simulink model "test_qr4_est"  (Simulink 7.0)
settings: Solver=ode45  StartTime=0.0  StopTime=10.0  RelTol=1e-3
libraries: xbsIndex_r4 x1048
(part 1 of 18)
settings Model: Creator=homin  LastModifiedBy=homin
settings DebuggingCC: SaveWithParameterizedLinksMsg=none  SignalResolutionControl=TryResolveAllWithWarning  MultiTaskDSMMsg=warning  MultiTaskCondExecSysMsg=none  StrictBusMsg=None
settings RTWCC: IncludeERTFirstTime=on
settings GRTTargetCC: TargetFcnLib=ansi_tfl_tmw.mat

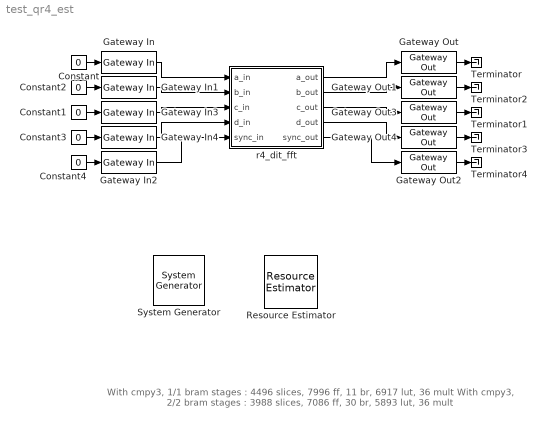
== system test_qr4_est ==
  note: With cmpy3, 1/1 bram stages : 4496 slices, 7996 ff, 11 br, 6917 lut, 36 mult
      | With cmpy3, 2/2 bram stages : 3988 slices, 7086 ff, 30 br, 5893 lut, 36 mult
  " System Generator" : xbsIndex_r4/ System Generator  Tag=genX  SystemSampleTime=-1  xilinxfamily=Virtex2P  part=xc2vp40  speed=-6  package=ff1152  synthesis_tool=XST  clock_wrapper=Clock Enables  directory=./test_qr4_est.netlist  testbench=off  simulink_period=1  sysclk_period=10  dcm_input_clock_period=100  incr_netlist=off  trim_vbits=Everywhere in SubSystem  dbl_ovrd=According to Block Masks  core_generation=According to Block Masks  run_coregen=off  deprecated_control=off  eval_field=0  block_type=sysgen
      settings: block_version=10.1.3
  Constant{,1..4} (5 alike) : Constant  Value=0  OutDataType=sfix(16)  OutScaling=2^0
  Gateway In{,1,3..4} (4 alike) : xbsIndex_r4/Gateway In  arith_type=Unsigned  n_bits=16  bin_pt=0  quantization=Truncate  overflow=Wrap  period=1  dbl_ovrd=off  timing_constraint=None  locs_specified=off  LOCs={}  block_type=gatewayin
      settings: infoedit="Gateway in block.  Converts inputs of type Simulink integer, double and fixed point to  Xilinx fixed point type.<P><P>Hardware notes:  In hardware these blocks become top level input ports."  xl_area=[0 0 0 0 16 0 0]  block_version=10.1.3
  Gateway In2 : xbsIndex_r4/Gateway In  arith_type=Boolean  n_bits=8  bin_pt=6  quantization=Truncate  overflow=Wrap  period=1  dbl_ovrd=off  timing_constraint=None  locs_specified=off  LOCs={}  block_type=gatewayin
      settings: infoedit="Gateway in block.  Converts inputs of type Simulink integer, double and fixed point to  Xilinx fixed point type.<P><P>Hardware notes:  In hardware these blocks become top level input ports."  xl_area=[0 0 0 0 1 0 0]  block_version=10.1.3
  Gateway Out{,1..4} (5 alike) : xbsIndex_r4/Gateway Out  hdl_port=on  timing_constraint=None  locs_specified=off  LOCs={}  block_type=gatewayout
      Gateway Out settings: infoedit="Gateway out block.  Converts Xilinx fixed point inputs into ouputs of type Simulink integer, double, or fixed point.<P><P>Hardware notes:  In hardware these blocks become top level output ports or are discarded, depending on how they are configured."  xl_area=[0 0 0 0 36 0 0]  block_version=10.1.3
      Gateway Out1 settings: infoedit="Gateway out block.  Converts Xilinx fixed point inputs into ouputs of type Simulink integer, double, or fixed point.<P><P>Hardware notes:  In hardware these blocks become top level output ports or are discarded, depending on how they are configured."  xl_area=[0 0 0 0 36 0 0]  block_version=10.1.3
      Gateway Out2 settings: infoedit="Gateway out block.  Converts Xilinx fixed point inputs into ouputs of type Simulink integer, double, or fixed point.<P><P>Hardware notes:  In hardware these blocks become top level output ports or are discarded, depending on how they are configured."  xl_area=[0 0 0 0 1 0 0]  block_version=10.1.3
      Gateway Out3 settings: infoedit="Gateway out block.  Converts Xilinx fixed point inputs into ouputs of type Simulink integer, double, or fixed point.<P><P>Hardware notes:  In hardware these blocks become top level output ports or are discarded, depending on how they are configured."  xl_area=[0 0 0 0 36 0 0]  block_version=10.1.3
      Gateway Out4 settings: infoedit="Gateway out block.  Converts Xilinx fixed point inputs into ouputs of type Simulink integer, double, or fixed point.<P><P>Hardware notes:  In hardware these blocks become top level output ports or are discarded, depending on how they are configured."  xl_area=[0 0 0 0 36 0 0]  block_version=10.1.3
  Resource Estimator : xbsIndex_r4/Resource Estimator  Tag=resEstTag  Slices=4588  FFs=5908  BRAMs=11  LUTs=6917  IOBs=210  EBMs=36  TBUFs=0  xl_use_estimator_area=off  est_options=Estimate  xl_estimator_area=[4496 7996 11 6917 210 36 0]  mrp_directory=./test_qr4_est.netlist  simulink_period=1  block_type=resource_estimator
      settings: AttributesFormatString=Resource Estimator\n%<xl_estimator_area>\n[SL FF BR LUT IO MUL TBUF]  block_version=10.1.3
  Terminator{,1..4} (5 alike) : Terminator
  r4_dit_fft : Subsystem  AncestorBlock=newfft_library/FFT/r4_dit_fft  mask(Quadplex Radix-4 DIT FFT){n_stages=5, n_bits=8, bin_pt=7, shifts=[0], commutator_bram=1, twiddle_bram=1, n_bits_w=9, mult_latency=3, add_latency=1, commute_output=No, output_order=Bit Reversed, show_sbo=on, munge_submasks=DumbDown}
      mask prompts: n_stages "Total Stages"; n_bits "Number of Bits In"; bin_pt "Binary Point In"; shifts "Shifting Schedule"; commutator_bram "Number of Stages Using BRAM for Biplex Commutators (i.e. delays)"; twiddle_bram "Number of Stages Using BRAM for Twiddle Coefficients"; n_bits_w "Twiddle Coefficient Bitwidth"; mult_latency "Multiplier Latency"; add_latency "Adder Latency"; commute_output "Commute Output"; output_order "Output Order"; show_sbo "Show Sub-Block Options"; munge_submasks "Sub-Block Masks"
      mask help: A quadplex radix-4 decimation-in-time Fast Fourier Transform.
      mask init:
      | tic
      | r4_dit_fft_init(gcb, ...
      |   n_stages, ...
      |   n_bits, ...
      |   bin_pt, ...
      |   shifts, ...
      |   commutator_bram, ...
      |   twiddle_bram, ...
      |   n_bits_w, ...
      |   mult_latency, ...
      |   add_latency, ...
      |   commute_output, ...
      |   output_order, ...
      |   lower(get_param(gcb,'munge_submasks')) );
      | disp('r4_dit_fft initialization complete.');
      | toc
      settings: AttributesFormatString=|
      | 1024 points
      | 8_7 r/i in
      | 9_7 twiddles
      mask Help:
      | <pre>
      | Description::
      | 
      | A quadplex radix-4 decimation-in-time Fast Fourier Transform.
      | 
      | The four inputs to the quadplex FFT are independent complex signals (e.g. A, B, C, D).
      | 
      | Without an output commutator, the four outputs of the FFT are commuted such that the
      | a_out signal is really the first quarter of A's transform followed by the first quarter of B's
      | transform, the first quarter of C's transform and the first quarter of D's transform.
      | b_out is really the seconds quarter of A's transform followed by the second quarter of
      | B's transform and so on for the rest of b_out as well as c_out and d_out.
      | 
      | If it is desired to have the four quarters of A's transform follow each other on the
      | same path (and so on for the transforms of B, C, and D), then be sure to check the
      | "Output Commutator" checkbox.  This will result in the four quarters of A's transform
      | (or B's, C's, D's) being in sequential order.  Including the output commutator uses additional
      | resources.
      | 
      | If the Normal Ouput Order option is chosen, the output will be in normal order (though still in
      | commuted quarters if no output commutator is used).  If the "Bit Reversed" Output Order"
      | option is selected, the output quarters (either commuted or not) will each be in bit reversed
      | order (i.e. each quarter of each transform will be in bit reversed output order).   Normal output
      | is easier for humans to work with (especially for testing), but it uses additional resources.
      | Bit reversed output is the implementation's inhernet output order so that option uses no
      | additional resources.
      | 
      | 
      | The number of bits for each real and imaginary component grows by two through this stage.
      | If the bit width grows to exceed 17 bits (when using three real multiplies per complex multiply;
      | 18 bits when using 4 real multiplies per complex multiply), then subsequent stages will
      | comsume more FPGA resources.  A future version will provide an option to limit bit growth.
      | 
      | The number of bits for each real and imaginary component grows by two through each stage.
      | If a stage's input bit width is 17 or less, three embedded multipliers will be used per complex multiply.
      | If a stage's input bit width is 18, four embedded multipliers will be used per complex multiply.
      | If a stage's input bit width exceeds 18, then substantially more embedded multipliers will be used
      | per complex multiply.  Enabling "shifting" in some (or all) stages can limit the bit growth
      | to prevent this.  See the Shifting Schedule parameter for more info.
      | 
      | 
      | Mask Parameters::
      | 
      | Total Stages (n_stages):  The number of total stages in the FFT.
      | The FFT will have 4^n_stages points.
      | 
      | Number of Bits In (n_bits): Specifies the width of the real/imaginary components of ports
      | a_in and b_in.  Assumed equal for both components.  The output bit width will be
      | n_bits+2*n_stages (assuming sum(shifts)==0).
      | 
      | Binary Point In/Out (bin_pt): Specifies the binary point position of the real/imaginary
      | components of ports a_in, b_in, c_in, and d_in.  Assumed equal for both components.
      | 
      | Shifting Schedule (shifts): A vector specifying how many bits to shift by at each stage.
      | Missing values are assumed to be zero; extra values are ignored.
      | 
      | Number of Stages Using BRAM for Biplex Commutators (commutator_bram): Number of stages
      | that will use BRAM for commutator memory.  Remaining stages will use SLR16 elements (slices).
      | 
      | Number of Stages Using BRAM for Twiddle Coefficients (twiddle_bram): Number of stages that
      | will use BRAM for twiddle coeeficient storage.  Remaining stages will use distributed memory
      | (slices).
      | 
      | Twiddle Coefficient Bitwidth (n_bits_w): Specifies the width of the real/imaginary
      | components of the twiddle coefficients.  Assumed equal for both components.
      | 
      | Multiplier Latency (mult_latency): Latency to use for the underlying real multipliers.
      | 
      | Adder Latency (add_latency): Latency to use for the underlying real adders.
      | 
      | Commute Output (commute_output): Popup options for an output commutator.  See decription
      | above for details on the output commutator.  Choices are:
      |     "No" - No output commutator
      |     "Yes (SLR16)" - Include output commutator using SLR16 elements
      |     "Yes (BRAM)" - Include output commutator using BRAM
      | 
      | Output Order (output_order): Popup options for selecting the output order.  See description
      | above for details on the output order.  Choices are:
      |     "Bit Reversed" - Output each half of each transform in bit reversed order.
      |     "Normal" - Output each half of each transform in normal order.
      | </pre>
      mask StyleString: edit,edit,edit,edit,edit,edit,edit,edit,edit,popup(No|Yes (SLR16)|Yes (BRAM)),popup(Bit Reversed|Normal),checkbox,popup(Keep|DumbDown|Unmask)
      mask CallbackString:
      | |||||||||||mvs=get_param(gcb,'MaskVisibilityString');
      | if strcmp(get_param(gcb,'show_sbo'),'on')
      |   onoff='on';
      | else
      |   onoff='off';
      | end
      | mvs=regexprep(mvs,'o[nf]*$',onoff);
      | set_param(gcb,'MaskVisibilityString',mvs);
      | |
  wires:
  Gateway In/1 -> r4_dit_fft/1(a_in)
  r4_dit_fft/1(a_out) -> Gateway Out/1
  Gateway In1/1 -> r4_dit_fft/2(b_in)
  Gateway In2/1 -> r4_dit_fft/5(sync_in)
  r4_dit_fft/2(b_out) -> Gateway Out1/1
  r4_dit_fft/5(sync_out) -> Gateway Out2/1
  Constant/1 -> Gateway In/1
  Constant2/1 -> Gateway In1/1
  Constant4/1 -> Gateway In2/1
  Gateway Out/1 -> Terminator/1
  Gateway Out1/1 -> Terminator2/1
  Gateway Out2/1 -> Terminator4/1
  Gateway In3/1 -> r4_dit_fft/3(c_in)
  Gateway In4/1 -> r4_dit_fft/4(d_in)
  Constant1/1 -> Gateway In3/1
  Constant3/1 -> Gateway In4/1
  r4_dit_fft/3(c_out) -> Gateway Out3/1
  r4_dit_fft/4(d_out) -> Gateway Out4/1
  Gateway Out3/1 -> Terminator1/1
  Gateway Out4/1 -> Terminator3/1

== system test_qr4_est/r4_dit_fft ==
  a_in : Inport  OutDataType=sfix(16)  OutScaling=2^0
  b_in : Inport  Port=2  OutDataType=sfix(16)  OutScaling=2^0
  c_in : Inport  Port=3  OutDataType=sfix(16)  OutScaling=2^0
  d_in : Inport  Port=4  OutDataType=sfix(16)  OutScaling=2^0
  sync_in : Inport  Port=5  OutDataType=sfix(16)  OutScaling=2^0
  r4_dit_stage_1 : Subsystem  mask(Radix-4 DIT FFT Stage){n_stages=5, cur_stage=1, n_bits=8, bin_pt=7, shift=0, commutator_bram=on, twiddle_bram=off, n_bits_w=9, mult_latency=3, add_latency=1}
      mask prompts: n_stages "Total Stages (4^N points)"; cur_stage "Current Stage"; n_bits "Number of Bits In"; bin_pt "Binary Point In"; shift "Shift Bits"; commutator_bram "Use BRAM for Quadplex Commutator"; twiddle_bram "Use BRAM for Twiddle Coefficients"; n_bits_w "Twiddle Coefficient Bitwidth"; mult_latency "Multiplier Latency"; add_latency "Adder Latency"
      mask help: A radix-4 decimation-in-time Fast Fourier Transform stage.
      settings: AttributesFormatString=|
      | stage 1 of 5
      | delay bram
      | twiddle dist
      | shift 0
      mask Help:
      | <pre>
      | Description::
      | 
      | A radix-4 decimation-in-time Fast Fourier Transform stage.
      | 
      | This radix-4 decimation-in-time FFT stage is designed to be daisy chained together
      | to form a multi-stage FFT.  The resulting FFT will have (4^n_stages) points.
      | 
      | The four inputs to the chain are independent complex signals (e.g. A, B, C, and D).
      | 
      | The four outputs of the last stage of the chain are commuted such that the a_out signal is really
      | the first quarter of A's transform followed by the first quarter of B's transform, the first quarter
      | of C's transform and the first quarter of D's transform.  b_out is really the seconds quarter of
      | A's transform followed by the second quarter of B's transform and so on for the rest of b_out
      | as well as c_out and d_out.  Each quarter is in bit-reversed order.
      | 
      | If it is desired to have the four quarters of A's transform follow each other on the
      | same path (and so on for the transforms of B, C, and D), then a_out and b_out can
      | be fed through a quadplex_commutator with block size 4^n_stages.  This will result
      | in the four quarters of A's transform (or B's, C's, D's) being in sequential order,
      | but note that each quarter of A's transform will still remain in bit-reversed order
      | (i.e. each output is bit-reversed in quarterss; it is not bit reversed in its entirety).
      | 
      | The number of bits for each real and imaginary component grows by two through this stage.
      | If the input bit width is 17 or less, three embedded multipliers will be used per complex multiply.
      | If the input bit width is 18, four embedded multipliers will be used per complex multiply.
      | If the input bit width exceeds 18, then substantially more embedded multipliers will be used
      | per complex multiply.  Enabling "shifting" in some (or all) stages can limit the bit growth
      | to prevent this.
      | 
      | Mask Parameters::
      | 
      | Total Stages (n_stages):  The number of total stages in the FFT.
      | The FFT will have 4^n_stages points.
      | 
      | Current Stage (cur_stage):  The number of the current stage.  Note that stages are counted
      | from 1 to n_stages for DIT (i.e. cur_stage==1 for the first stage).
      | 
      | Number of Bits In (n_bits): Specifies the width of the real/imaginary components of ports
      | a_in and b_in.  Assumed equal for both components.  The real/imaginary components of
      | oorts a_out and b_out will be one bit wider.
      | 
      | Binary Point In (bin_pt): Specifies the binary point position of the real/imaginary
      | components of ports a_in and b_in.  Assumed equal for both components.
      | 
      | Shift Bits (shift): Specifies how many bits to shift (down) by.  A positive value causes
      | the specified number of least significant bits to be dropped.  Usually zero or positive values
      | are used to permit or limit bit growth, but negative values can be used to induce bit growth.
      | 
      | Use BRAM for Biplex Commutator (commutator_bram): Check this checkbox to implement
      | the biplex commutator using BRAM.  If unchecked, the biplex commutator will be implemented
      | using SLR16 elements (i.e. slices).
      | 
      | Use BRAM for Twiddle Coefficients (twiddle_bram): Check this checkbox to store twiddle
      | coefficients in BRAM.  If unchecked, the twiddle coefficients will be sored in distributed
      | memory (i.e. slices).
      | 
      | Twiddle Coefficient Bitwidth (n_bits_w): Specifies the width of the real/imaginary
      | components of the twiddle coefficients.  Assumed equal for both components.
      | 
      | Multiplier Latency (mult_latency): Latency to use for the underlying real multipliers.
      | 
      | Adder Latency (add_latency): Latency to use for the underlying real adders.
      | </pre>
  r4_dit_stage_2 : Subsystem  mask(Radix-4 DIT FFT Stage){n_stages=5, cur_stage=2, n_bits=10, bin_pt=7, shift=0, commutator_bram=off, twiddle_bram=off, n_bits_w=9, mult_latency=3, add_latency=1}
      mask prompts: n_stages "Total Stages (4^N points)"; cur_stage "Current Stage"; n_bits "Number of Bits In"; bin_pt "Binary Point In"; shift "Shift Bits"; commutator_bram "Use BRAM for Quadplex Commutator"; twiddle_bram "Use BRAM for Twiddle Coefficients"; n_bits_w "Twiddle Coefficient Bitwidth"; mult_latency "Multiplier Latency"; add_latency "Adder Latency"
      mask help: A radix-4 decimation-in-time Fast Fourier Transform stage.
      settings: AttributesFormatString=|
      | stage 2 of 5
      | delay slr
      | twiddle dist
      | shift 0
      mask Help:
      | <pre>
      | Description::
      | 
      | A radix-4 decimation-in-time Fast Fourier Transform stage.
      | 
      | This radix-4 decimation-in-time FFT stage is designed to be daisy chained together
      | to form a multi-stage FFT.  The resulting FFT will have (4^n_stages) points.
      | 
      | The four inputs to the chain are independent complex signals (e.g. A, B, C, and D).
      | 
      | The four outputs of the last stage of the chain are commuted such that the a_out signal is really
      | the first quarter of A's transform followed by the first quarter of B's transform, the first quarter
      | of C's transform and the first quarter of D's transform.  b_out is really the seconds quarter of
      | A's transform followed by the second quarter of B's transform and so on for the rest of b_out
      | as well as c_out and d_out.  Each quarter is in bit-reversed order.
      | 
      | If it is desired to have the four quarters of A's transform follow each other on the
      | same path (and so on for the transforms of B, C, and D), then a_out and b_out can
      | be fed through a quadplex_commutator with block size 4^n_stages.  This will result
      | in the four quarters of A's transform (or B's, C's, D's) being in sequential order,
      | but note that each quarter of A's transform will still remain in bit-reversed order
      | (i.e. each output is bit-reversed in quarterss; it is not bit reversed in its entirety).
      | 
      | The number of bits for each real and imaginary component grows by two through this stage.
      | If the input bit width is 17 or less, three embedded multipliers will be used per complex multiply.
      | If the input bit width is 18, four embedded multipliers will be used per complex multiply.
      | If the input bit width exceeds 18, then substantially more embedded multipliers will be used
      | per complex multiply.  Enabling "shifting" in some (or all) stages can limit the bit growth
      | to prevent this.
      | 
      | Mask Parameters::
      | 
      | Total Stages (n_stages):  The number of total stages in the FFT.
      | The FFT will have 4^n_stages points.
      | 
      | Current Stage (cur_stage):  The number of the current stage.  Note that stages are counted
      | from 1 to n_stages for DIT (i.e. cur_stage==1 for the first stage).
      | 
      | Number of Bits In (n_bits): Specifies the width of the real/imaginary components of ports
      | a_in and b_in.  Assumed equal for both components.  The real/imaginary components of
      | oorts a_out and b_out will be one bit wider.
      | 
      | Binary Point In (bin_pt): Specifies the binary point position of the real/imaginary
      | components of ports a_in and b_in.  Assumed equal for both components.
      | 
      | Shift Bits (shift): Specifies how many bits to shift (down) by.  A positive value causes
      | the specified number of least significant bits to be dropped.  Usually zero or positive values
      | are used to permit or limit bit growth, but negative values can be used to induce bit growth.
      | 
      | Use BRAM for Biplex Commutator (commutator_bram): Check this checkbox to implement
      | the biplex commutator using BRAM.  If unchecked, the biplex commutator will be implemented
      | using SLR16 elements (i.e. slices).
      | 
      | Use BRAM for Twiddle Coefficients (twiddle_bram): Check this checkbox to store twiddle
      | coefficients in BRAM.  If unchecked, the twiddle coefficients will be sored in distributed
      | memory (i.e. slices).
      | 
      | Twiddle Coefficient Bitwidth (n_bits_w): Specifies the width of the real/imaginary
      | components of the twiddle coefficients.  Assumed equal for both components.
      | 
      | Multiplier Latency (mult_latency): Latency to use for the underlying real multipliers.
      | 
      | Adder Latency (add_latency): Latency to use for the underlying real adders.
      | </pre>
  r4_dit_stage_3 : Subsystem  mask(Radix-4 DIT FFT Stage){n_stages=5, cur_stage=3, n_bits=12, bin_pt=7, shift=0, commutator_bram=off, twiddle_bram=off, n_bits_w=9, mult_latency=3, add_latency=1}
      mask prompts: n_stages "Total Stages (4^N points)"; cur_stage "Current Stage"; n_bits "Number of Bits In"; bin_pt "Binary Point In"; shift "Shift Bits"; commutator_bram "Use BRAM for Quadplex Commutator"; twiddle_bram "Use BRAM for Twiddle Coefficients"; n_bits_w "Twiddle Coefficient Bitwidth"; mult_latency "Multiplier Latency"; add_latency "Adder Latency"
      mask help: A radix-4 decimation-in-time Fast Fourier Transform stage.
      settings: AttributesFormatString=|
      | stage 3 of 5
      | delay slr
      | twiddle dist
      | shift 0
      mask Help:
      | <pre>
      | Description::
      | 
      | A radix-4 decimation-in-time Fast Fourier Transform stage.
      | 
      | This radix-4 decimation-in-time FFT stage is designed to be daisy chained together
      | to form a multi-stage FFT.  The resulting FFT will have (4^n_stages) points.
      | 
      | The four inputs to the chain are independent complex signals (e.g. A, B, C, and D).
      | 
      | The four outputs of the last stage of the chain are commuted such that the a_out signal is really
      | the first quarter of A's transform followed by the first quarter of B's transform, the first quarter
      | of C's transform and the first quarter of D's transform.  b_out is really the seconds quarter of
      | A's transform followed by the second quarter of B's transform and so on for the rest of b_out
      | as well as c_out and d_out.  Each quarter is in bit-reversed order.
      | 
      | If it is desired to have the four quarters of A's transform follow each other on the
      | same path (and so on for the transforms of B, C, and D), then a_out and b_out can
      | be fed through a quadplex_commutator with block size 4^n_stages.  This will result
      | in the four quarters of A's transform (or B's, C's, D's) being in sequential order,
      | but note that each quarter of A's transform will still remain in bit-reversed order
      | (i.e. each output is bit-reversed in quarterss; it is not bit reversed in its entirety).
      | 
      | The number of bits for each real and imaginary component grows by two through this stage.
      | If the input bit width is 17 or less, three embedded multipliers will be used per complex multiply.
      | If the input bit width is 18, four embedded multipliers will be used per complex multiply.
      | If the input bit width exceeds 18, then substantially more embedded multipliers will be used
      | per complex multiply.  Enabling "shifting" in some (or all) stages can limit the bit growth
      | to prevent this.
      | 
      | Mask Parameters::
      | 
      | Total Stages (n_stages):  The number of total stages in the FFT.
      | The FFT will have 4^n_stages points.
      | 
      | Current Stage (cur_stage):  The number of the current stage.  Note that stages are counted
      | from 1 to n_stages for DIT (i.e. cur_stage==1 for the first stage).
      | 
      | Number of Bits In (n_bits): Specifies the width of the real/imaginary components of ports
      | a_in and b_in.  Assumed equal for both components.  The real/imaginary components of
      | oorts a_out and b_out will be one bit wider.
      | 
      | Binary Point In (bin_pt): Specifies the binary point position of the real/imaginary
      | components of ports a_in and b_in.  Assumed equal for both components.
      | 
      | Shift Bits (shift): Specifies how many bits to shift (down) by.  A positive value causes
      | the specified number of least significant bits to be dropped.  Usually zero or positive values
      | are used to permit or limit bit growth, but negative values can be used to induce bit growth.
      | 
      | Use BRAM for Biplex Commutator (commutator_bram): Check this checkbox to implement
      | the biplex commutator using BRAM.  If unchecked, the biplex commutator will be implemented
      | using SLR16 elements (i.e. slices).
      | 
      | Use BRAM for Twiddle Coefficients (twiddle_bram): Check this checkbox to store twiddle
      | coefficients in BRAM.  If unchecked, the twiddle coefficients will be sored in distributed
      | memory (i.e. slices).
      | 
      | Twiddle Coefficient Bitwidth (n_bits_w): Specifies the width of the real/imaginary
      | components of the twiddle coefficients.  Assumed equal for both components.
      | 
      | Multiplier Latency (mult_latency): Latency to use for the underlying real multipliers.
      | 
      | Adder Latency (add_latency): Latency to use for the underlying real adders.
      | </pre>
  r4_dit_stage_4 : Subsystem  mask(Radix-4 DIT FFT Stage){n_stages=5, cur_stage=4, n_bits=14, bin_pt=7, shift=0, commutator_bram=off, twiddle_bram=off, n_bits_w=9, mult_latency=3, add_latency=1}
      mask prompts: n_stages "Total Stages (4^N points)"; cur_stage "Current Stage"; n_bits "Number of Bits In"; bin_pt "Binary Point In"; shift "Shift Bits"; commutator_bram "Use BRAM for Quadplex Commutator"; twiddle_bram "Use BRAM for Twiddle Coefficients"; n_bits_w "Twiddle Coefficient Bitwidth"; mult_latency "Multiplier Latency"; add_latency "Adder Latency"
      mask help: A radix-4 decimation-in-time Fast Fourier Transform stage.
      settings: AttributesFormatString=|
      | stage 4 of 5
      | delay slr
      | twiddle dist
      | shift 0
      mask Help:
      | <pre>
      | Description::
      | 
      | A radix-4 decimation-in-time Fast Fourier Transform stage.
      | 
      | This radix-4 decimation-in-time FFT stage is designed to be daisy chained together
      | to form a multi-stage FFT.  The resulting FFT will have (4^n_stages) points.
      | 
      | The four inputs to the chain are independent complex signals (e.g. A, B, C, and D).
      | 
      | The four outputs of the last stage of the chain are commuted such that the a_out signal is really
      | the first quarter of A's transform followed by the first quarter of B's transform, the first quarter
      | of C's transform and the first quarter of D's transform.  b_out is really the seconds quarter of
      | A's transform followed by the second quarter of B's transform and so on for the rest of b_out
      | as well as c_out and d_out.  Each quarter is in bit-reversed order.
      | 
      | If it is desired to have the four quarters of A's transform follow each other on the
      | same path (and so on for the transforms of B, C, and D), then a_out and b_out can
      | be fed through a quadplex_commutator with block size 4^n_stages.  This will result
      | in the four quarters of A's transform (or B's, C's, D's) being in sequential order,
      | but note that each quarter of A's transform will still remain in bit-reversed order
      | (i.e. each output is bit-reversed in quarterss; it is not bit reversed in its entirety).
      | 
      | The number of bits for each real and imaginary component grows by two through this stage.
      | If the input bit width is 17 or less, three embedded multipliers will be used per complex multiply.
      | If the input bit width is 18, four embedded multipliers will be used per complex multiply.
      | If the input bit width exceeds 18, then substantially more embedded multipliers will be used
      | per complex multiply.  Enabling "shifting" in some (or all) stages can limit the bit growth
      | to prevent this.
      | 
      | Mask Parameters::
      | 
      | Total Stages (n_stages):  The number of total stages in the FFT.
      | The FFT will have 4^n_stages points.
      | 
      | Current Stage (cur_stage):  The number of the current stage.  Note that stages are counted
      | from 1 to n_stages for DIT (i.e. cur_stage==1 for the first stage).
      | 
      | Number of Bits In (n_bits): Specifies the width of the real/imaginary components of ports
      | a_in and b_in.  Assumed equal for both components.  The real/imaginary components of
      | oorts a_out and b_out will be one bit wider.
      | 
      | Binary Point In (bin_pt): Specifies the binary point position of the real/imaginary
      | components of ports a_in and b_in.  Assumed equal for both components.
      | 
      | Shift Bits (shift): Specifies how many bits to shift (down) by.  A positive value causes
      | the specified number of least significant bits to be dropped.  Usually zero or positive values
      | are used to permit or limit bit growth, but negative values can be used to induce bit growth.
      | 
      | Use BRAM for Biplex Commutator (commutator_bram): Check this checkbox to implement
      | the biplex commutator using BRAM.  If unchecked, the biplex commutator will be implemented
      | using SLR16 elements (i.e. slices).
      | 
      | Use BRAM for Twiddle Coefficients (twiddle_bram): Check this checkbox to store twiddle
      | coefficients in BRAM.  If unchecked, the twiddle coefficients will be sored in distributed
      | memory (i.e. slices).
      | 
      | Twiddle Coefficient Bitwidth (n_bits_w): Specifies the width of the real/imaginary
      | components of the twiddle coefficients.  Assumed equal for both components.
      | 
      | Multiplier Latency (mult_latency): Latency to use for the underlying real multipliers.
      | 
      | Adder Latency (add_latency): Latency to use for the underlying real adders.
      | </pre>
  r4_dit_stage_5 : Subsystem  mask(Radix-4 DIT FFT Stage){n_stages=5, cur_stage=5, n_bits=16, bin_pt=7, shift=0, commutator_bram=off, twiddle_bram=on, n_bits_w=9, mult_latency=3, add_latency=1}
      mask prompts: n_stages "Total Stages (4^N points)"; cur_stage "Current Stage"; n_bits "Number of Bits In"; bin_pt "Binary Point In"; shift "Shift Bits"; commutator_bram "Use BRAM for Quadplex Commutator"; twiddle_bram "Use BRAM for Twiddle Coefficients"; n_bits_w "Twiddle Coefficient Bitwidth"; mult_latency "Multiplier Latency"; add_latency "Adder Latency"
      mask help: A radix-4 decimation-in-time Fast Fourier Transform stage.
      settings: AttributesFormatString=|
      | stage 5 of 5
      | delay slr
      | twiddle bram
      | shift 0
      mask Help:
      | <pre>
      | Description::
      | 
      | A radix-4 decimation-in-time Fast Fourier Transform stage.
      | 
      | This radix-4 decimation-in-time FFT stage is designed to be daisy chained together
      | to form a multi-stage FFT.  The resulting FFT will have (4^n_stages) points.
      | 
      | The four inputs to the chain are independent complex signals (e.g. A, B, C, and D).
      | 
      | The four outputs of the last stage of the chain are commuted such that the a_out signal is really
      | the first quarter of A's transform followed by the first quarter of B's transform, the first quarter
      | of C's transform and the first quarter of D's transform.  b_out is really the seconds quarter of
      | A's transform followed by the second quarter of B's transform and so on for the rest of b_out
      | as well as c_out and d_out.  Each quarter is in bit-reversed order.
      | 
      | If it is desired to have the four quarters of A's transform follow each other on the
      | same path (and so on for the transforms of B, C, and D), then a_out and b_out can
      | be fed through a quadplex_commutator with block size 4^n_stages.  This will result
      | in the four quarters of A's transform (or B's, C's, D's) being in sequential order,
      | but note that each quarter of A's transform will still remain in bit-reversed order
      | (i.e. each output is bit-reversed in quarterss; it is not bit reversed in its entirety).
      | 
      | The number of bits for each real and imaginary component grows by two through this stage.
      | If the input bit width is 17 or less, three embedded multipliers will be used per complex multiply.
      | If the input bit width is 18, four embedded multipliers will be used per complex multiply.
      | If the input bit width exceeds 18, then substantially more embedded multipliers will be used
      | per complex multiply.  Enabling "shifting" in some (or all) stages can limit the bit growth
      | to prevent this.
      | 
      | Mask Parameters::
      | 
      | Total Stages (n_stages):  The number of total stages in the FFT.
      | The FFT will have 4^n_stages points.
      | 
      | Current Stage (cur_stage):  The number of the current stage.  Note that stages are counted
      | from 1 to n_stages for DIT (i.e. cur_stage==1 for the first stage).
      | 
      | Number of Bits In (n_bits): Specifies the width of the real/imaginary components of ports
      | a_in and b_in.  Assumed equal for both components.  The real/imaginary components of
      | oorts a_out and b_out will be one bit wider.
      | 
      | Binary Point In (bin_pt): Specifies the binary point position of the real/imaginary
      | components of ports a_in and b_in.  Assumed equal for both components.
      | 
      | Shift Bits (shift): Specifies how many bits to shift (down) by.  A positive value causes
      | the specified number of least significant bits to be dropped.  Usually zero or positive values
      | are used to permit or limit bit growth, but negative values can be used to induce bit growth.
      | 
      | Use BRAM for Biplex Commutator (commutator_bram): Check this checkbox to implement
      | the biplex commutator using BRAM.  If unchecked, the biplex commutator will be implemented
      | using SLR16 elements (i.e. slices).
      | 
      | Use BRAM for Twiddle Coefficients (twiddle_bram): Check this checkbox to store twiddle
      | coefficients in BRAM.  If unchecked, the twiddle coefficients will be sored in distributed
      | memory (i.e. slices).
      | 
      | Twiddle Coefficient Bitwidth (n_bits_w): Specifies the width of the real/imaginary
      | components of the twiddle coefficients.  Assumed equal for both components.
      | 
      | Multiplier Latency (mult_latency): Latency to use for the underlying real multipliers.
      | 
      | Adder Latency (add_latency): Latency to use for the underlying real adders.
      | </pre>
  a_out : Outport  OutDataType=sfix(16)  OutScaling=2^0
  b_out : Outport  Port=2  OutDataType=sfix(16)  OutScaling=2^0
  c_out : Outport  Port=3  OutDataType=sfix(16)  OutScaling=2^0
  d_out : Outport  Port=4  OutDataType=sfix(16)  OutScaling=2^0
  sync_out : Outport  Port=5  OutDataType=sfix(16)  OutScaling=2^0
  wires:
  a_in/1 -> r4_dit_stage_1/1(a_in)
  b_in/1 -> r4_dit_stage_1/2(b_in)
  c_in/1 -> r4_dit_stage_1/3(c_in)
  d_in/1 -> r4_dit_stage_1/4(d_in)
  sync_in/1 -> r4_dit_stage_1/5(sync_in)
  r4_dit_stage_1/1(a_out) -> r4_dit_stage_2/1(a_in)
  r4_dit_stage_1/2(b_out) -> r4_dit_stage_2/2(b_in)
  r4_dit_stage_1/3(c_out) -> r4_dit_stage_2/3(c_in)
  r4_dit_stage_1/4(d_out) -> r4_dit_stage_2/4(d_in)
  r4_dit_stage_1/5(sync_out) -> r4_dit_stage_2/5(sync_in)
  r4_dit_stage_2/1(a_out) -> r4_dit_stage_3/1(a_in)
  r4_dit_stage_2/2(b_out) -> r4_dit_stage_3/2(b_in)
  r4_dit_stage_2/3(c_out) -> r4_dit_stage_3/3(c_in)
  r4_dit_stage_2/4(d_out) -> r4_dit_stage_3/4(d_in)
  r4_dit_stage_2/5(sync_out) -> r4_dit_stage_3/5(sync_in)
  r4_dit_stage_3/1(a_out) -> r4_dit_stage_4/1(a_in)
  r4_dit_stage_3/2(b_out) -> r4_dit_stage_4/2(b_in)
  r4_dit_stage_3/3(c_out) -> r4_dit_stage_4/3(c_in)
  r4_dit_stage_3/4(d_out) -> r4_dit_stage_4/4(d_in)
  r4_dit_stage_3/5(sync_out) -> r4_dit_stage_4/5(sync_in)
  r4_dit_stage_4/1(a_out) -> r4_dit_stage_5/1(a_in)
  r4_dit_stage_4/2(b_out) -> r4_dit_stage_5/2(b_in)
  r4_dit_stage_4/3(c_out) -> r4_dit_stage_5/3(c_in)
  r4_dit_stage_4/4(d_out) -> r4_dit_stage_5/4(d_in)
  r4_dit_stage_4/5(sync_out) -> r4_dit_stage_5/5(sync_in)
  r4_dit_stage_5/1(a_out) -> a_out/1
  r4_dit_stage_5/3(c_out) -> b_out/1
  r4_dit_stage_5/2(b_out) -> c_out/1
  r4_dit_stage_5/4(d_out) -> d_out/1
  r4_dit_stage_5/5(sync_out) -> sync_out/1

== system test_qr4_est/r4_dit_fft/r4_dit_stage_1 ==
  a_in : Inport  OutDataType=sfix(16)  OutScaling=2^0
  b_in : Inport  Port=2  OutDataType=sfix(16)  OutScaling=2^0
  c_in : Inport  Port=3  OutDataType=sfix(16)  OutScaling=2^0
  d_in : Inport  Port=4  OutDataType=sfix(16)  OutScaling=2^0
  sync_in : Inport  Port=5  OutDataType=sfix(16)  OutScaling=2^0
  quadplex_commutator : Subsystem  mask(Quadplex Commutator){log4_size=5, n_bits=8, use_bram=on}
      mask prompts: log4_size "Log4 Block Size"; n_bits "Bit Width"; use_bram "Use BRAM"
      mask help: The quadplex commutator performs a "quarter-blockwise" commutation of the four inputs. A "block" is 4^log4_size consecutive samples (i.e. always a power of 4). sync_in precedes the first data input sample by one clock cycle. Overall latency from sync_in to sync_out is 2^(log4_size)+2^(log4_size-1)+2.
      settings: AttributesFormatString=|
      | size = 1024
      | 4/4 bram
      mask Help:
      | <pre>
      | Description::
      | 
      | The quadplex commutator performs a "quarter-blockwise" commutation of the four inputs.
      | A "block" is 4^log4_size consecutive samples (i.e. always a power of 4).
      | 
      | sync_in precedes the first data input sample by one clock cycle.
      | sync_out precedes the corresponding output sample by one clock cycle.
      | Overall latency from sync_in to sync_out is 2^(log4_size)+2^(log4_size-1)+2.
      | 
      | Mask Parameters::
      | 
      | Log4 Block Size (log4_size): The base-4 logarithm of the length of one complete input block.
      | This MUST be an integer because the current implementation requires that
      | the input block size MUST be a power of 4.  (aka "N")
      | 
      | Bit Width (n_bits): Specifies the width of the real/imaginary components.
      | Width of each component is assumed equal.
      | 
      | Use BRAM (use_bram): Check this checkbox to implement the internal delays using BRAM.
      | If unchecked, the internal delays will be implemented using SLR16 elements.
      | </pre>
  r4_butterfly : Subsystem  mask(Radix-4 Butterfly){n_bits=8, shift=0, quantization=Truncate, add_latency=1}
      mask prompts: n_bits "Bit Width In"; shift "Shift Bits"; add_latency "Adder Latency"
      mask help: The radix-4 butterfly performs a 4 point FFT on its four inputs (a_in,b_in,c_in,d_in), which are assumed to be in normal order. Its ouputs (a_out,b_out,c_out,d_out) are in bit-reversed order (despite the lexigraphical ordering of the output port names).
      settings: AttributesFormatString=shift 0
      mask Help:
      | <pre>
      | Description::
      | 
      | The radix-4 butterfly performs a 4 point FFT on its four inputs (a_in,b_in,c_in,d_in),
      | which are assumed to be in normal order.  Its ouputs (a_out,b_out,c_out,d_out) are
      | in bit-reversed order (despite the lexigraphical ordering of the output port names).
      | 
      | The outputs are two bits wider than the inputs.
      | The output precision (i.e. the number of fractional bits) stays the same.
      | 
      | Mask Parameters::
      | 
      | Bit Width In (n_bits): Specifies the width of the real/imaginary components.
      | Width of each component is assumed equal.
      | 
      | Shift Bits (shift): Specifies how many bits to shift (down) by.  A positive value causes
      | the specified number of least significant bits to be dropped.  Usually zero or positive values
      | are used to permit or limit bit growth, but negative values can be used to induce bit growth.
      | 
      | Quantization (quantization): Specifies quantization handling (when shift bits > 0).
      | 
      | Adder Latency (add_latency): Latency to use for the underlying real adders.
      | </pre>
      mask StyleString: edit,edit,popup(Truncate|Round  (unbiased: +/- Inf)|Round  (unbiased: Even Values)),edit
  r4_twiddle : Subsystem
      mask Type: Radix-4 Stage-1 Twiddle Stage
      mask Description: A stage-1 twiddle stage for radix-4 Fast Fourier Transforms. Since there are no twiddles in stage 1 of an FFT, this is just a dummy placeholder block that passes its inputs through to its outputs.    Since it is a no-op, its use is completely optional.
      mask Help:
      | <pre>
      | Description::
      | 
      | A stage-1 twiddle stage for radix-4 Fast Fourier Transforms.
      | 
      | Since there are no twiddles in stage 1 of an FFT, this is just a dummy placeholder
      | block that passes its inputs through to its outputs.
      | 
      | Since it is a no-op, its use is completely optional.
      | 
      | Note that stages are counted from 1 to n_stages for DIT (i.e. cur_stage==1 for the first stage)
      | and n_stages to 1for DIF (i.e. cur_stage==1 for the last stage).  Therefore, this block, if used,
      | should be the first twiddle stage of a DIT FFT or the last twiddle stage of a DIF FFT.
      | 
      | Mask Parameters::
      | 
      | (N/A)
  a_out : Outport  OutDataType=sfix(16)  OutScaling=2^0
  b_out : Outport  Port=2  OutDataType=sfix(16)  OutScaling=2^0
  c_out : Outport  Port=3  OutDataType=sfix(16)  OutScaling=2^0
  d_out : Outport  Port=4  OutDataType=sfix(16)  OutScaling=2^0
  sync_out : Outport  Port=5  OutDataType=sfix(16)  OutScaling=2^0
  wires:
  r4_butterfly/5(sync_out) -> sync_out/1
  r4_butterfly/4(d_out) -> d_out/1
  r4_butterfly/3(c_out) -> c_out/1
  r4_butterfly/2(b_out) -> b_out/1
  r4_butterfly/1(a_out) -> a_out/1
  sync_in/1 -> quadplex_commutator/5(sync_in)
  d_in/1 -> quadplex_commutator/4(d)
  c_in/1 -> quadplex_commutator/3(c)
  b_in/1 -> quadplex_commutator/2(b)
  a_in/1 -> quadplex_commutator/1(a)
  r4_twiddle/5(sync_out) -> r4_butterfly/5(sync_in)
  r4_twiddle/4(d_out) -> r4_butterfly/4(d_in)
  r4_twiddle/3(c_out) -> r4_butterfly/3(c_in)
  r4_twiddle/2(b_out) -> r4_butterfly/2(b_in)
  r4_twiddle/1(a_out) -> r4_butterfly/1(a_in)
  quadplex_commutator/5(sync_out) -> r4_twiddle/5(sync_in)
  quadplex_commutator/4(abcd3) -> r4_twiddle/4(d_in)
  quadplex_commutator/3(abcd2) -> r4_twiddle/3(c_in)
  quadplex_commutator/2(abcd1) -> r4_twiddle/2(b_in)
  quadplex_commutator/1(abcd0) -> r4_twiddle/1(a_in)
